simulink model "sUASTrajectoryStates"  (R2021b)
settings: Solver=VariableStepAuto  StartTime=0.0  StopTime=900  RelTol=1e-3
InitFcn:
  | FidelityStage = 2;
model workspace (MAT data in the model file):
  AirspeedVal = 58.2251893932
  LookaheadDc = 50
  LookaheadDistance = 500
  Waypoints = [-5313.43403732 -5313.49765579 -5315.24259606 -5316.98751886 -5318.73267892 -5320.47705726 -5322.22141779 -5323.96550555 -5324.69997396 -5326.29075872 -5327.88101514 -5329.47150848 ... (2598 elements, 866x3)]
  airspeedVal = 34.4977795798
  headingAngles : timeseries (value not decoded)
  lookaheadPoint : timeseries (value not decoded)
  waypointData = [-1625.03275672 -1598.86938118 -1571.45340762 -1543.27035087 -1514.50729286 -1485.12594864 -1455.09042939 -1424.58849905 -1393.84251756 -1362.78862848 -1331.63098268 -1300.4045263 ... (291 elements, 97x3)]
undefined symbols (not defined in the file): aircraftTmax, ap, DiscIntNeverNeededParam, Earth, env, initialThrottle, midFidelityUAV, sensors, trimT, uavParam, WGS84
libraries: simulink x21, mbdriLib x20, aerolibconvert2 x2, aerolibtransform2 x1, uavalgslib x1
(part 2 of 3)

== system sUASTrajectoryStates/Heading to Bank Angle ==
  TargetHeading : Inport  OutDataTypeStr=double  PortDimensions=1
  Environment : Inport  Port=2
  State : Inport  Port=3
  Bus Selector : BusSelector  OutputSignals=AirSpeed,HeadingAngle,FlightPathAngle
  Bus Selector1 : BusSelector  OutputSignals=WindNorth,WindEast,WindDown,Gravity
  HeadingControllerGain : Constant  Value=4.88135593220339  SampleTime=0.1
  Limit Bank to +- 45 deg : Saturate  UpperLimit=midFidelityUAV.maxroll/180*pi  LowerLimit=-midFidelityUAV.maxroll/180*pi
  MATLAB Function : MATLAB Function  TreatAsAtomicUnit=on
  TargetMu : Outport
  wires:
  Limit Bank to +- 45 deg/1 -> TargetMu/1  "BankAngle"
  Bus Selector1/4 -> MATLAB Function/8(Gravity)  "<Gravity>"
  Bus Selector1/3 -> MATLAB Function/7(WindDown)  "<WindDown>"
  Bus Selector1/2 -> MATLAB Function/6(WindEast)  "<WindEast>"
  Bus Selector1/1 -> MATLAB Function/5(WindNorth)  "<WindNorth>"
  TargetHeading/1 -> MATLAB Function/4(TargetHeading)
  Bus Selector/2 -> MATLAB Function/2(HeadingAngle)  "<HeadingAngle>"
  Bus Selector/1 -> MATLAB Function/1(AirSpeed)  "<AirSpeed>"
  Environment/1 -> Bus Selector1/1
  State/1 -> Bus Selector/1
  HeadingControllerGain/1 -> MATLAB Function/9(PHeadingAngle)
  Bus Selector/3 -> MATLAB Function/3(FlightPathAngle)  "<FlightPathAngle>"
  MATLAB Function/1(RollAngle) -> Limit Bank to +- 45 deg/1

== system sUASTrajectoryStates/uavEnvironment ==
  note: Gravity and Density ASSUME MKS units!
  note: Steady wind vector components (m/s).
      | (WindNorth is not from the North, as in meteorology,
      | but the component in the Northerly direction.)
  Bus Creator : BusCreator  Inputs=5
  Constant1 : Constant  Value=0
  Constant2 : Constant  Value=0
  Constant3 : Constant  Value=0
  g : Constant  Value=9.8066
  rho : Constant  Value=1.225
  SteadyEnvironment : Outport  VectorParamsAs1DForOutWhenUnconnected=off
  wires:
  Constant2/1 -> Bus Creator/2  "WindEast"
  Constant3/1 -> Bus Creator/3  "WindDown"
  Constant1/1 -> Bus Creator/1  "WindNorth"
  Bus Creator/1 -> SteadyEnvironment/1
  g/1 -> Bus Creator/4  "Gravity"
  rho/1 -> Bus Creator/5  "Density"

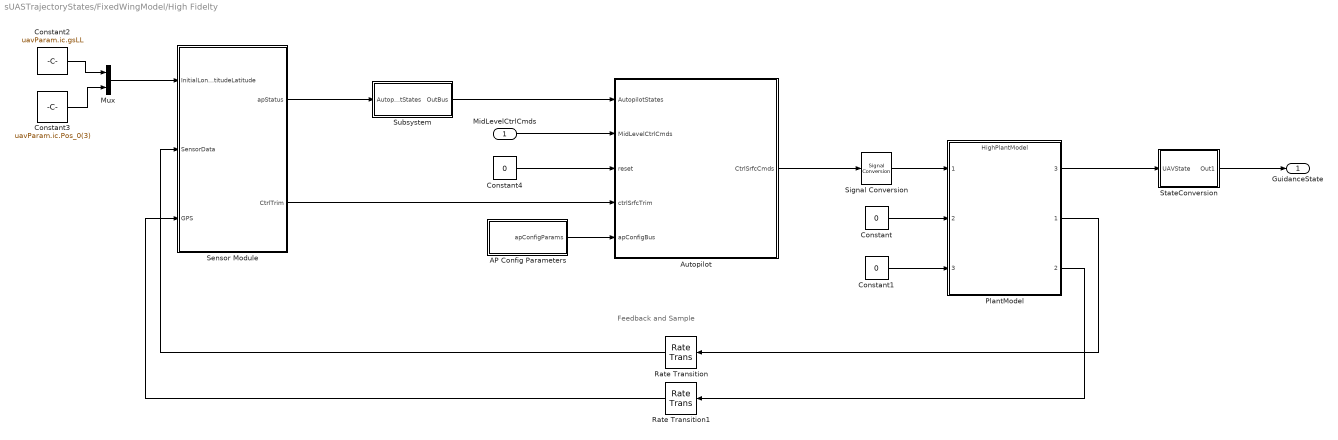
== system sUASTrajectoryStates/FixedWingModel/High Fidelty ==
  note: Feedback and Sample
  MidLevelCtrlCmds : Inport
  AP Config Parameters : Subsystem
  Autopilot : Subsystem
  Constant : Constant  Value=0
  Constant1 : Constant  Value=0
  Constant2 : Constant  Value=uavParam.ic.gsLL  OutDataTypeStr=single
  Constant3 : Constant  Value=uavParam.ic.Pos_0(3)  OutDataTypeStr=single
  Constant4 : Constant  Value=0
  Mux : Mux  Inputs=2
  PlantModel : ModelReference  ModelNameDialog=HighPlantModel.slx  SimulationMode=Normal  ModelReferenceVersion=2.0
      settings: PortSchema="{\"entries\":[{\"content\":{\"sides\":[{\"content\":{\"connectorIds\":[\"In1\",\"In2\",\"In3\"]},\"type\":\"ConnectorPlacement.EquallySpacedRectSide\",\"uuid\":\"b05064ba-762f-4c47-8c4a-e4b5b8698203\"},{\"content\":{\"connectorIds\":[\"Out3\",\"Out1\",\"Out2\"],\"side\":\"RIGHT\"},\"type\":\"ConnectorPlacement.EquallySpacedRectSide\",\"uuid\":\"4dd868b9-025c-4261-91c2-75e76041d933\"},{\"content\":{\"connectorIds\":[],\"side\":\"TOP\"},\"type\":\"ConnectorPlacement.EquallySpacedRectSide\",\"uuid\":\"bfb2a469-2e8b-4568-a482-f0d58a8ec089\"}]},\"type\":\"ConnectorPlacement.EquallySpacedConnector\",\"uuid\":\"89fe167c-302c-412e-9468-047389136680\"}],\"packageUris\":[\"http://schema.mathworks.com/mf0/Connector/R2020b\"],\"version\":\"1.0\"}"
  Rate Transition : RateTransition  OutPortSampleTime=ap.apSampleTime
  Rate Transition1 : RateTransition  OutPortSampleTime=ap.apSampleTime
      settings: AttributesFormatString=%<OutPortSampleTime>
  Sensor Module : Subsystem
  Signal Conversion : SignalConversion  ConversionOutput=Nonvirtual bus  OutDataTypeStr=Bus: ctrlCmdsBus  OverrideOpt=off
  StateConversion : Subsystem
  Subsystem : Subsystem
  GuidanceState : Outport
  wires:
  PlantModel/1 -> Rate Transition/1
  PlantModel/3 -> StateConversion/1(UAVState)
  StateConversion/1(Out1) -> GuidanceState/1
  Mux/1 -> Sensor Module/1(InitialLongtitudeLatitude)
  Constant2/1 -> Mux/1
  Constant1/1 -> PlantModel/3
  Constant/1 -> PlantModel/2
  PlantModel/2 -> Rate Transition1/1
  Constant3/1 -> Mux/2
  Rate Transition/1 -> Sensor Module/2(SensorData)
  Rate Transition1/1 -> Sensor Module/3(GPS)
  Signal Conversion/1 -> PlantModel/1
  Sensor Module/1(apStatus) -> Subsystem/1(AutopilotStates)
  Subsystem/1(OutBus) -> Autopilot/1(AutopilotStates)
  MidLevelCtrlCmds/1 -> Autopilot/2(MidLevelCtrlCmds)
  Constant4/1 -> Autopilot/3(reset)
  Sensor Module/2(CtrlTrim) -> Autopilot/4(ctrlSrfcTrim)
  AP Config Parameters/1(apConfigParams) -> Autopilot/5(apConfigBus)
  Autopilot/1(CtrlSrfcCmds) -> Signal Conversion/1

== system sUASTrajectoryStates/FixedWingModel/LowFidelity ==
  MidLevelCtrlCmds : Inport
  Bus Creator1 : BusCreator  Inputs=4  OutDataTypeStr=Bus: FixedWingEnvironmentBus  NonVirtualBus=on
  Constant : Constant  Value=0
  Constant1 : Constant  Value=0
  Constant2 : Constant  Value=0
  Constant5 : Constant  Value=env.ISA_g
  Fixed Wing UAV Guidance Model : uavalgslib/Guidance Model  ModelType=FixedWingGuidance  SpecifiedDataType=double  SimulateUsing=Code generation  InitialWorldPositionMultirotor=[0; 0; 0]  InitialWorldVelocityMultirotor=[0; 0; 0]  InitialEulerZYXMultirotor=[0; 0; 0]  InitialBodyAngularRateRPYMultirotor=[0; 0; 0]  InitialThrustMultirotor=0  InitialNorthFixedWing=0  InitialEastFixedWing=0  InitialHeightFixedWing=lowFidelityUAV.initialAltitude  InitialAirSpeedFixedWing=lowFidelityUAV.initialAirSpeed  InitialHeadingAngleFixedWing=0  InitialFlightPathAngleFixedWing=0  InitialRollAngleFixedWing=0  InitialRollAngleRateFixedWing=0  PDRollMultirotor=[3402.97,116.67]  PDPitchMultirotor=[3402.97, 116.67]  PYawRateMultirotor=1950  PThrustMultirotor=3900  MassMultirotor=0.1  PHeightFixedWing=3  PHeadingAngleFixedWing=3.9  PFlightPathAngleFixedWing=3.9  PDRollFixedWing="[5.448     4.6668]"  PAirSpeedFixedWing=7.8  FlightPathAngleLimitsFixedWing=[-pi/4, pi/4]  StateBusName='FixedWingStateBus'  ControlBusName='FixedWingControlBus'  EnvironmentBusName='FixedWingEnvironmentBus'  DataType=double
      settings: SourceProductBaseCode=UV
  GuidanceState : Outport  VectorParamsAs1DForOutWhenUnconnected=off
  wires:
  Constant5/1 -> Bus Creator1/4  "Gravity"
  Constant1/1 -> Bus Creator1/2  "WindEast"
  Bus Creator1/1 -> Fixed Wing UAV Guidance Model/2
  MidLevelCtrlCmds/1 -> Fixed Wing UAV Guidance Model/1
  Constant/1 -> Bus Creator1/1  "WindNorth"
  Fixed Wing UAV Guidance Model/1 -> GuidanceState/1
  Constant2/1 -> Bus Creator1/3  "WindDown"

== system sUASTrajectoryStates/FixedWingModel/Mid Fidelty ==
  MidLevelCtrlCmds : Inport
  Constant : Constant  Value=0
  Delay : Delay  DelayLength=1  InitialCondition=struct('Xe', [0 0 midFidelityUAV.initialAltitude], 'ias',midFidelityUAV.initialAirspeed)  SampleTime=ap.apSampleTime
  Model : ModelReference  ModelNameDialog=Outer_Loop_Autopilot.slx  SimulationMode=Normal  ModelReferenceVersion=2.10
  Rate Transition1 : RateTransition  OutPortSampleTime=0.1
  UAV Plant Dynamics : Subsystem  TreatAsAtomicUnit=on
  uavEnvironment : Subsystem  VariantControl=NoWind
  GuidanceState : Outport
  wires:
  uavEnvironment/1(SteadyEnvironment) -> UAV Plant Dynamics/2(Environment)
  Model/1 -> UAV Plant Dynamics/1(Commands)
  UAV Plant Dynamics/2(AutopilotStates) -> Rate Transition1/1
  UAV Plant Dynamics/1(uavState) -> GuidanceState/1
  Delay/1 -> Model/1
  MidLevelCtrlCmds/1 -> Model/2
  Rate Transition1/1 -> Delay/1
  Constant/1 -> Model/3

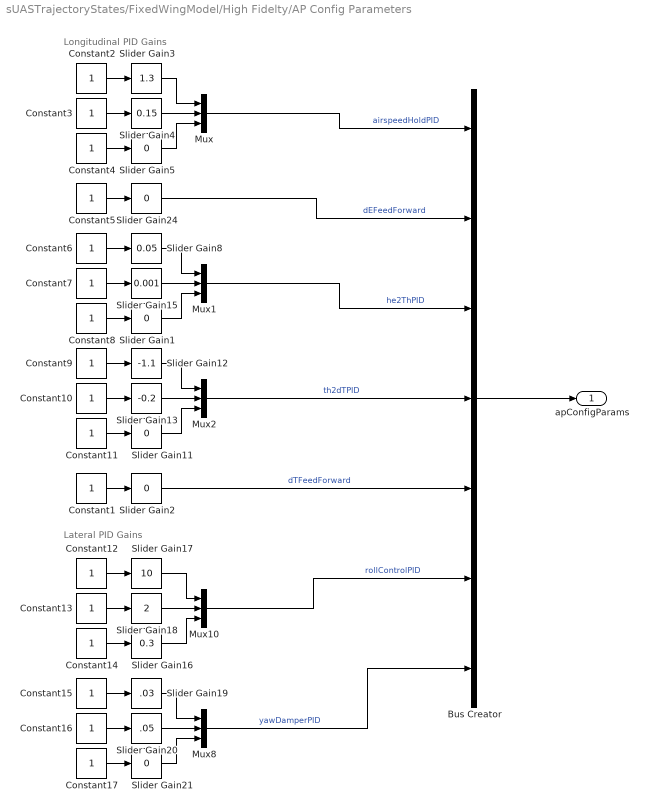
== system sUASTrajectoryStates/FixedWingModel/High Fidelty/AP Config Parameters ==
  note: Longitudinal PID Gains
  note: Lateral PID Gains
  Bus Creator : BusCreator  Inputs=7  OutDataTypeStr=Bus: apConfigParamsBus
  Constant{1..17} (17 alike) : Constant  OutDataTypeStr=single  SampleTime=ap.apSampleTime
      settings: AttributesFormatString=%<Value>
  Mux{,1..2,8,10} (5 alike) : Mux  Inputs=3
  Slider Gain1 : simulink/Math Operations/Slider Gain  gain=0  low=-20  high=20
  Slider Gain11 : simulink/Math Operations/Slider Gain  gain=0  low=-0.1  high=0
  Slider Gain12 : simulink/Math Operations/Slider Gain  gain=-1.1  low=-2  high=0.5
  Slider Gain13 : simulink/Math Operations/Slider Gain  gain=-0.2  low=-0.2  high=0
  Slider Gain15 : simulink/Math Operations/Slider Gain  gain=0.001  low=-20  high=20
  Slider Gain16 : simulink/Math Operations/Slider Gain  gain=0.3  low=-0.1  high=5
  Slider Gain17 : simulink/Math Operations/Slider Gain  gain=10  low=-0.1  high=50
  Slider Gain18 : simulink/Math Operations/Slider Gain  gain=2  low=0  high=2
  Slider Gain19 : simulink/Math Operations/Slider Gain  gain=.03  low=-20  high=20
  Slider Gain2 : simulink/Math Operations/Slider Gain  gain=0  low=-0.1  high=5
  Slider Gain20 : simulink/Math Operations/Slider Gain  gain=.05  low=-20  high=20
  Slider Gain21 : simulink/Math Operations/Slider Gain  gain=0  low=-20  high=20
  Slider Gain24 : simulink/Math Operations/Slider Gain  gain=0  low=-0.1  high=5
  Slider Gain3 : simulink/Math Operations/Slider Gain  gain=1.3  low=-0.5  high=4.5
  Slider Gain4 : simulink/Math Operations/Slider Gain  gain=0.15  low=-20  high=20
  Slider Gain5 : simulink/Math Operations/Slider Gain  gain=0  low=-20  high=20
  Slider Gain8 : simulink/Math Operations/Slider Gain  gain=0.05  low=-20  high=20
  apConfigParams : Outport  OutDataTypeStr=Bus: apConfigParamsBus  VectorParamsAs1DForOutWhenUnconnected=off
  wires:
  Mux8/1 -> Bus Creator/7  "yawDamperPID"
  Slider Gain21/1 -> Mux8/3
  Slider Gain19/1 -> Mux8/1
  Slider Gain20/1 -> Mux8/2
  Constant17/1 -> Slider Gain21/1
  Constant16/1 -> Slider Gain20/1
  Constant15/1 -> Slider Gain19/1
  Mux10/1 -> Bus Creator/6  "rollControlPID"
  Slider Gain16/1 -> Mux10/3
  Slider Gain17/1 -> Mux10/1
  Slider Gain18/1 -> Mux10/2
  Constant14/1 -> Slider Gain16/1
  Constant13/1 -> Slider Gain18/1
  Constant12/1 -> Slider Gain17/1
  Constant1/1 -> Slider Gain2/1
  Slider Gain1/1 -> Mux1/3
  Slider Gain15/1 -> Mux1/2
  Mux2/1 -> Bus Creator/4  "th2dTPID"
  Slider Gain11/1 -> Mux2/3
  Slider Gain12/1 -> Mux2/1
  Slider Gain13/1 -> Mux2/2
  Constant11/1 -> Slider Gain11/1
  Constant10/1 -> Slider Gain13/1
  Constant9/1 -> Slider Gain12/1
  Mux1/1 -> Bus Creator/3  "he2ThPID"
  Slider Gain8/1 -> Mux1/1
  Constant8/1 -> Slider Gain1/1
  Constant7/1 -> Slider Gain15/1
  Constant6/1 -> Slider Gain8/1
  Slider Gain24/1 -> Bus Creator/2  "dEFeedForward"
  Constant5/1 -> Slider Gain24/1
  Mux/1 -> Bus Creator/1  "airspeedHoldPID"
  Slider Gain5/1 -> Mux/3
  Slider Gain3/1 -> Mux/1
  Slider Gain4/1 -> Mux/2
  Constant4/1 -> Slider Gain5/1
  Constant3/1 -> Slider Gain4/1
  Constant2/1 -> Slider Gain3/1
  Bus Creator/1 -> apConfigParams/1
  Slider Gain2/1 -> Bus Creator/5  "dTFeedForward"

== system sUASTrajectoryStates/FixedWingModel/High Fidelty/Autopilot ==
  note: Signal Routing
  AutopilotStates : Inport
  MidLevelCtrlCmds : Inport  Port=2
  reset : Inport  Port=3
  ctrlSrfcTrim : Inport  Port=4
  apConfigBus : Inport  Port=5
  Inner Loop Autopilot : Subsystem
  Outer Loop Autopilot : ModelReference  ModelNameDialog=Outer_Loop_Autopilot.slx  SimulationMode=Normal  ModelReferenceVersion=2.6
      settings: PortSchema="{\"entries\":[{\"content\":{\"sides\":[{\"content\":{\"connectorIds\":[\"In2\",\"In1\",\"In3\"]},\"type\":\"ConnectorPlacement.EquallySpacedRectSide\",\"uuid\":\"ffbe0e68-5eaf-4f2c-bade-2815524b0984\"},{\"content\":{\"connectorIds\":[\"Out1\"],\"side\":\"RIGHT\"},\"type\":\"ConnectorPlacement.EquallySpacedRectSide\",\"uuid\":\"57fe3717-6620-4a33-be9b-5bc5f2cad269\"},{\"content\":{\"connectorIds\":[],\"side\":\"TOP\"},\"type\":\"ConnectorPlacement.EquallySpacedRectSide\",\"uuid\":\"35a1b882-87be-41ec-998f-2c84a3803ec5\"}]},\"type\":\"ConnectorPlacement.EquallySpacedConnector\",\"uuid\":\"d728f9c7-d9da-4786-9d89-76839d7f2fee\"}],\"packageUris\":[\"http://schema.mathworks.com/mf0/Connector/R2020b\"],\"version\":\"1.0\"}"
  CtrlSrfcCmds : Outport
  wires:
  Inner Loop Autopilot/1(CtrlSrfcCmds) -> CtrlSrfcCmds/1
  [AutopilotStates] -> Outer Loop Autopilot/1
  MidLevelCtrlCmds/1 -> Outer Loop Autopilot/2
  apConfigBus/1 -> Inner Loop Autopilot/5(apConfigBus)
  Outer Loop Autopilot/1 -> Inner Loop Autopilot/1(LowLevelCtrlCmds)
  ctrlSrfcTrim/1 -> Inner Loop Autopilot/4(ctrlSrfcTrim)
  AutopilotStates/1 -> [AutopilotStates]
  reset/1 -> [reset]
  [AutopilotStates] -> Inner Loop Autopilot/2(AutopilotStates)
  [reset] -> Inner Loop Autopilot/3(reset)
  [reset] -> Outer Loop Autopilot/3

== system sUASTrajectoryStates/FixedWingModel/High Fidelty/Sensor Module ==
  InitialLongtitudeLatitude : Inport
  SensorData : Inport  Port=2
  GPS : Inport  Port=3
  Position Filter : Subsystem  TreatAsAtomicUnit=on
  SensorConditioning : Subsystem  TreatAsAtomicUnit=on
  apStatusCreation : Subsystem
  apStatus : Outport  VectorParamsAs1DForOutWhenUnconnected=off
  CtrlTrim : Outport  Port=2  VectorParamsAs1DForOutWhenUnconnected=off
  wires:
  InitialLongtitudeLatitude/1 -> Position Filter/3(InitialLongtitudeLatitude)
  SensorConditioning/1(FilteredSensorData) -> apStatusCreation/3(FilteredSensorData), Position Filter/1(FilteredSensorData)
  SensorConditioning/2(CtrlSurfaces) -> CtrlTrim/1
  GPS/1 -> apStatusCreation/2(GPSData), Position Filter/2(GPSData)
  SensorData/1 -> SensorConditioning/1(RawSensorData)
  apStatusCreation/1(apStatus) -> apStatus/1
  Position Filter/1(PosVel_hat) -> apStatusCreation/1(PosVel_hat)

== system sUASTrajectoryStates/FixedWingModel/High Fidelty/StateConversion ==
  UAVState : Inport
  Bus Creator : BusCreator  Inputs=8  OutDataTypeStr=Bus: FixedWingStateBus  NonVirtualBus=on
  Bus Selector : BusSelector  OutputSignals=X_e,airspeed,V_e,Euler,pqr
  Demux : Demux  Outputs=3
  Gain : Gain  Gain=-1
  Gain1 : Gain
  Selector : Selector  InputPortWidth=3  IndexOptions=Index vector (dialog)  Indices=[1]  OutputSizes=1
  Selector1 : Selector  InputPortWidth=3  IndexOptions=Index vector (dialog)  Indices=[1]  OutputSizes=1
  Subsystem : Subsystem
  Out1 : Outport  VectorParamsAs1DForOutWhenUnconnected=off
  wires:
  Bus Creator/1 -> Out1/1
  Gain1/1 -> Bus Creator/4  "AirSpeed"
  Subsystem/2(FlightPath) -> Bus Creator/6  "FlightPathAngle"
  Bus Selector/2 -> Gain1/1  "<airspeed>"
  Selector/1 -> Bus Creator/7  "RollAngle"
  Bus Selector/4 -> Selector/1  "<Euler>"
  Bus Selector/1 -> Demux/1  "<X_e>"
  Bus Selector/3 -> Subsystem/1(Ve)  "<V_e>"
  Demux/2 -> Bus Creator/2  "East"
  Bus Selector/5 -> Selector1/1  "<pqr>"
  Subsystem/1(Heading) -> Bus Creator/5  "HeadingAngle"
  Demux/1 -> Bus Creator/1  "North"
  Demux/3 -> Gain/1
  Selector1/1 -> Bus Creator/8  "RollAngleRate"
  Gain/1 -> Bus Creator/3  "Height"
  UAVState/1 -> Bus Selector/1

== system sUASTrajectoryStates/FixedWingModel/High Fidelty/Subsystem ==
  In Bus Element : Inport  PortName=AutopilotStates  Element=Ab
  In Bus Element2 : Inport  PortName=AutopilotStates  Element=Euler
  In Bus Element5 : Inport  PortName=AutopilotStates  Element=Xe
  In Bus Element4 : Inport  PortName=AutopilotStates  Element=ias
  Data Type Conversion{,2..3,5} (4 alike) : DataTypeConversion  OutDataTypeStr=double
  Out Bus Element : Outport  PortName=OutBus  Element=Ab
  Out Bus Element2 : Outport  PortName=OutBus  Element=Euler
  Out Bus Element4 : Outport  PortName=OutBus  Element=Xe
  Out Bus Element7 : Outport  PortName=OutBus  Element=ias
  wires:
  In Bus Element4/1 -> Data Type Conversion3/1  "ias"
  In Bus Element5/1 -> Data Type Conversion5/1  "Xe"
  In Bus Element2/1 -> Data Type Conversion2/1  "Euler"
  In Bus Element/1 -> Data Type Conversion/1  "Ab"
  Data Type Conversion/1 -> Out Bus Element/1
  Data Type Conversion2/1 -> Out Bus Element2/1
  Data Type Conversion3/1 -> Out Bus Element7/1
  Data Type Conversion5/1 -> Out Bus Element4/1

== system sUASTrajectoryStates/FixedWingModel/Mid Fidelty/UAV Plant Dynamics ==
  Commands : Inport
  Environment : Inport  Port=2
  Vehicle Dynamics : Subsystem
  asbState to uavState : Subsystem
  uavState : Outport
  AutopilotStates : Outport  Port=2
  wires:
  Vehicle Dynamics/1(AutopilotState) -> asbState to uavState/1(asbState), AutopilotStates/1
  asbState to uavState/1(uavState) -> uavState/1
  Commands/1 -> Vehicle Dynamics/1(Commands)
  Environment/1 -> Vehicle Dynamics/2(Environment)

== system sUASTrajectoryStates/FixedWingModel/Mid Fidelty/uavEnvironment ==
  note: Gravity and Density ASSUME MKS units!
  note: Steady wind vector components (m/s).
      | (WindNorth is not from the North, as in meteorology,
      | but the component in the Northerly direction.)
  Bus Creator : BusCreator  Inputs=5
  Constant1 : Constant  Value=0
  Constant2 : Constant  Value=0
  Constant3 : Constant  Value=0
  g : Constant  Value=9.8066
  rho : Constant  Value=1.225
  SteadyEnvironment : Outport  VectorParamsAs1DForOutWhenUnconnected=off
  wires:
  Constant2/1 -> Bus Creator/2  "WindEast"
  Constant3/1 -> Bus Creator/3  "WindDown"
  Constant1/1 -> Bus Creator/1  "WindNorth"
  Bus Creator/1 -> SteadyEnvironment/1
  g/1 -> Bus Creator/4  "Gravity"
  rho/1 -> Bus Creator/5  "Density"

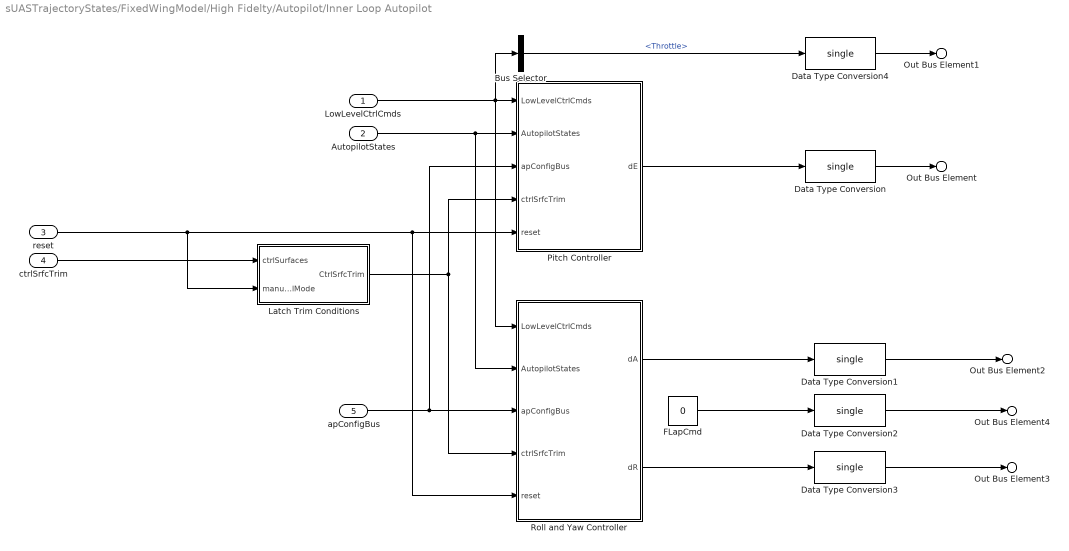
== system sUASTrajectoryStates/FixedWingModel/High Fidelty/Autopilot/Inner Loop Autopilot ==
  LowLevelCtrlCmds : Inport
  AutopilotStates : Inport  Port=2
  reset : Inport  Port=3
  ctrlSrfcTrim : Inport  Port=4
  apConfigBus : Inport  Port=5
  Bus Selector : BusSelector  OutputSignals=Throttle
  Data Type Conversion{,1..4} (5 alike) : DataTypeConversion  OutDataTypeStr=single
  FLapCmd : Constant  Value=0  OutDataTypeStr=single  SampleTime=ap.apSampleTime
      settings: AttributesFormatString=%<Value>
  Latch Trim Conditions : Subsystem
  Pitch Controller : Subsystem  VariantControl=AltCont==0
  Roll and Yaw Controller : Subsystem  TreatAsAtomicUnit=on
  Out Bus Element : Outport  PortName=CtrlSrfcCmds  Element=elevatorCmd
  Out Bus Element1 : Outport  PortName=CtrlSrfcCmds  Element=throttleCmd
  Out Bus Element2 : Outport  PortName=CtrlSrfcCmds  Element=aileronCmd
  Out Bus Element3 : Outport  PortName=CtrlSrfcCmds  Element=rudderCmd
  Out Bus Element4 : Outport  PortName=CtrlSrfcCmds  Element=flapCmd
  wires:
  Pitch Controller/1(dE) -> Data Type Conversion/1
  LowLevelCtrlCmds/1 -> Bus Selector/1, Roll and Yaw Controller/1(LowLevelCtrlCmds), Pitch Controller/1(LowLevelCtrlCmds)
  AutopilotStates/1 -> Roll and Yaw Controller/2(AutopilotStates), Pitch Controller/2(AutopilotStates)
  Latch Trim Conditions/1(CtrlSrfcTrim) -> Roll and Yaw Controller/4(ctrlSrfcTrim), Pitch Controller/4(ctrlSrfcTrim)
  Roll and Yaw Controller/1(dA) -> Data Type Conversion1/1
  Roll and Yaw Controller/2(dR) -> Data Type Conversion3/1
  apConfigBus/1 -> Pitch Controller/3(apConfigBus), Roll and Yaw Controller/3(apConfigBus)
  Bus Selector/1 -> Data Type Conversion4/1  "<Throttle>"
  ctrlSrfcTrim/1 -> Latch Trim Conditions/1(ctrlSurfaces)
  reset/1 -> Latch Trim Conditions/2(manualMode), Roll and Yaw Controller/5(reset), Pitch Controller/5(reset)
  Data Type Conversion/1 -> Out Bus Element/1
  Data Type Conversion1/1 -> Out Bus Element2/1
  FLapCmd/1 -> Data Type Conversion2/1
  Data Type Conversion2/1 -> Out Bus Element4/1
  Data Type Conversion3/1 -> Out Bus Element3/1
  Data Type Conversion4/1 -> Out Bus Element1/1

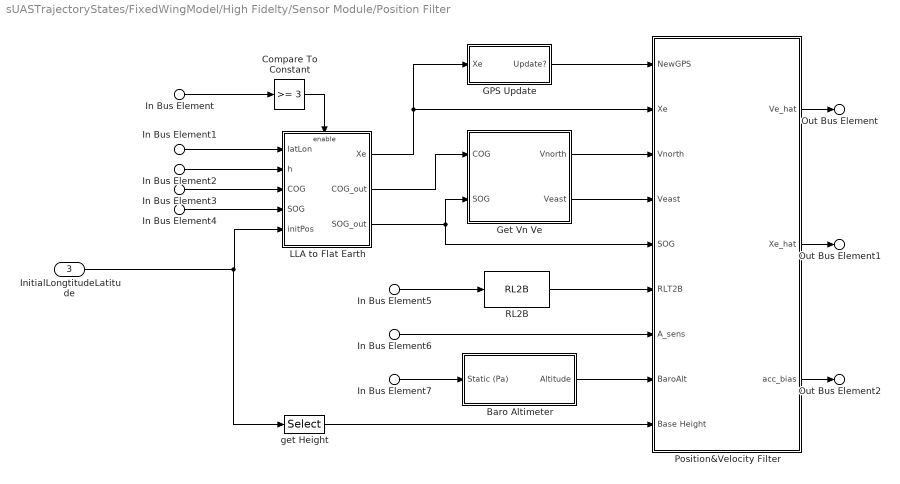
== system sUASTrajectoryStates/FixedWingModel/High Fidelty/Sensor Module/Position Filter ==
  In Bus Element5 : Inport  PortName=FilteredSensorData  Element=Euler
  In Bus Element6 : Inport  PortName=FilteredSensorData  Element=Ab
  In Bus Element7 : Inport  PortName=FilteredSensorData  Element=baro
  In Bus Element : Inport  Port=2  PortName=GPSData  Element=gps_fix
  In Bus Element1 : Inport  Port=2  PortName=GPSData  Element=gps_latLon
  In Bus Element2 : Inport  Port=2  PortName=GPSData  Element=gps_h
  In Bus Element3 : Inport  Port=2  PortName=GPSData  Element=gps_cog
  In Bus Element4 : Inport  Port=2  PortName=GPSData  Element=gps_sog
  InitialLongtitudeLatitude : Inport  Port=3
  Baro Altimeter : Subsystem
  Compare To Constant : simulink/Logic and Bit Operations/Compare To Constant  relop=>=  const=3  OutDataTypeStr=boolean
  GPS Update : Subsystem  mask{T=ap.apSampleTime}
      mask prompts: T "Sample Time"
  Get Vn Ve : Subsystem
  LLA to Flat Earth : Subsystem
  Position&Velocity Filter : Subsystem
  RL2B : mbdriLib/Coordinates/RL2B  SystemSampleTime=-1  VariantActivationTime=update diagram  Latency=0  AutoFrameSizeCalculation=off
  get Height : Selector  InputPortWidth=3  IndexOptions=Index vector (dialog)  Indices=[3]  OutputSizes=1
  Out Bus Element : Outport  VectorParamsAs1DForOutWhenUnconnected=off  PortName=PosVel_hat  Element=Ve_hat
  Out Bus Element1 : Outport  VectorParamsAs1DForOutWhenUnconnected=off  PortName=PosVel_hat  Element=Xe_hat
  Out Bus Element2 : Outport  VectorParamsAs1DForOutWhenUnconnected=off  PortName=PosVel_hat  Element=Ab_bias_hat
  wires:
  LLA to Flat Earth/1(Xe) -> Position&Velocity Filter/2(Xe), GPS Update/1(Xe)
  get Height/1 -> Position&Velocity Filter/9(Base Height)
  In Bus Element6/1 -> Position&Velocity Filter/7(A_sens)
  RL2B/1 -> Position&Velocity Filter/6(RLT2B)
  In Bus Element5/1 -> RL2B/1
  In Bus Element7/1 -> Baro Altimeter/1(Static (Pa))
  Baro Altimeter/1(Altitude) -> Position&Velocity Filter/8(BaroAlt)
  Get Vn Ve/2(Veast) -> Position&Velocity Filter/4(Veast)
  Get Vn Ve/1(Vnorth) -> Position&Velocity Filter/3(Vnorth)
  GPS Update/1(Update?) -> Position&Velocity Filter/1(NewGPS)
  InitialLongtitudeLatitude/1 -> LLA to Flat Earth/5(initPos), get Height/1
  In Bus Element4/1 -> LLA to Flat Earth/4(SOG)
  In Bus Element3/1 -> LLA to Flat Earth/3(COG)
  In Bus Element2/1 -> LLA to Flat Earth/2(h)
  In Bus Element1/1 -> LLA to Flat Earth/1(latLon)
  Compare To Constant/1 -> LLA to Flat Earth/Enable
  In Bus Element/1 -> Compare To Constant/1
  Position&Velocity Filter/2(Xe_hat) -> Out Bus Element1/1
  Position&Velocity Filter/1(Ve_hat) -> Out Bus Element/1
  Position&Velocity Filter/3(acc_bias) -> Out Bus Element2/1
  LLA to Flat Earth/2(COG_out) -> Get Vn Ve/1(COG)
  LLA to Flat Earth/3(SOG_out) -> Get Vn Ve/2(SOG), Position&Velocity Filter/5(SOG)

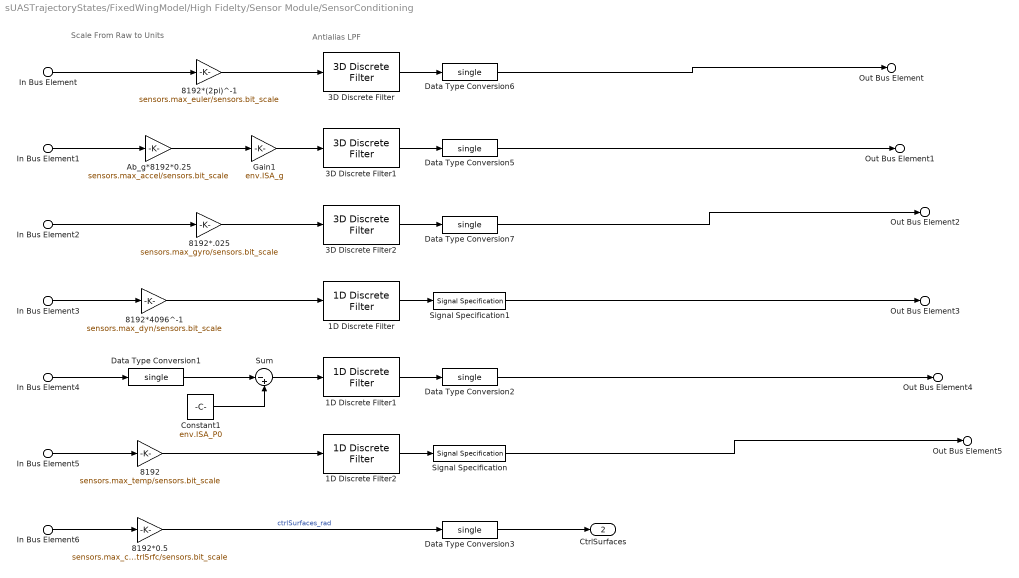
== system sUASTrajectoryStates/FixedWingModel/High Fidelty/Sensor Module/SensorConditioning ==
  note: Antialias LPF
  note: Scale From Raw to Units
  In Bus Element : Inport  PortName=RawSensorData  Element=Euler_raw
  In Bus Element1 : Inport  PortName=RawSensorData  Element=Ab_raw
  In Bus Element2 : Inport  PortName=RawSensorData  Element=G_raw
  In Bus Element3 : Inport  PortName=RawSensorData  Element=q_raw
  In Bus Element4 : Inport  PortName=RawSensorData  Element=static_raw
  In Bus Element5 : Inport  PortName=RawSensorData  Element=T_raw
  In Bus Element6 : Inport  PortName=RawSensorData  Element=ctrlSurface_PWM
  1D Discrete Filter : mbdriLib/Filtering/1D Discrete Filter  bw=sensors.antialiasBW  TSample=ap.apSampleTime
      settings: AttributesFormatString=Fc = 40
  1D Discrete Filter1 : mbdriLib/Filtering/1D Discrete Filter  bw=sensors.antialiasBW  TSample=ap.apSampleTime
      settings: AttributesFormatString=Fc = 40
  1D Discrete Filter2 : mbdriLib/Filtering/1D Discrete Filter  bw=sensors.antialiasBW  TSample=ap.apSampleTime
      settings: AttributesFormatString=Fc = 40
  3D Discrete Filter : mbdriLib/Filtering/3D Discrete Filter  bw=sensors.antialiasBW  TSample=ap.apSampleTime
      settings: AttributesFormatString=Fc = 40
  3D Discrete Filter1 : mbdriLib/Filtering/3D Discrete Filter  bw=sensors.antialiasBW  TSample=ap.apSampleTime
      settings: AttributesFormatString=Fc = 40
  3D Discrete Filter2 : mbdriLib/Filtering/3D Discrete Filter  bw=sensors.antialiasBW  TSample=ap.apSampleTime
      settings: AttributesFormatString=Fc = 40
  8192 : Gain  Description=8192/1  Gain=sensors.max_temp/sensors.bit_scale  OutDataTypeStr=single
      settings: AttributesFormatString=%<Gain>
  8192*(2pi)^-1 : Gain  Gain=sensors.max_euler/sensors.bit_scale  OutDataTypeStr=single
      settings: AttributesFormatString=%<Gain>
  8192*.025 : Gain  Gain=sensors.max_gyro/sensors.bit_scale  OutDataTypeStr=single
      settings: AttributesFormatString=%<Gain>
  8192*0.5 : Gain  Gain=sensors.max_ctrlSrfc/sensors.bit_scale  OutDataTypeStr=single
      settings: AttributesFormatString=%<Gain>
  8192*4096^-1 : Gain  Gain=sensors.max_dyn/sensors.bit_scale  OutDataTypeStr=single
      settings: AttributesFormatString=%<Gain>
  Ab_g*8192*0.25 : Gain  Gain=sensors.max_accel/sensors.bit_scale  OutDataTypeStr=single
      settings: AttributesFormatString=%<Gain>
  Constant1 : Constant  Value=env.ISA_P0
      settings: AttributesFormatString=%<Value>
  Data Type Conversion{1..3,5..7} (6 alike) : DataTypeConversion  OutDataTypeStr=single
  Gain1 : Gain  Gain=env.ISA_g  OutDataTypeStr=single
      settings: AttributesFormatString=%<Gain>
  Signal Specification : SignalSpecification  OutDataTypeStr=single  Unit=K
  Signal Specification1 : SignalSpecification  OutDataTypeStr=single  Unit=Pa
  Sum : Sum  Inputs=|-+
  Out Bus Element : Outport  VectorParamsAs1DForOutWhenUnconnected=off  PortName=FilteredSensorData  Element=Euler
  Out Bus Element1 : Outport  VectorParamsAs1DForOutWhenUnconnected=off  PortName=FilteredSensorData  Element=Ab
  Out Bus Element2 : Outport  VectorParamsAs1DForOutWhenUnconnected=off  PortName=FilteredSensorData  Element=G
  Out Bus Element3 : Outport  VectorParamsAs1DForOutWhenUnconnected=off  PortName=FilteredSensorData  Element=q
  Out Bus Element4 : Outport  VectorParamsAs1DForOutWhenUnconnected=off  PortName=FilteredSensorData  Element=baro
  Out Bus Element5 : Outport  VectorParamsAs1DForOutWhenUnconnected=off  PortName=FilteredSensorData  Element=T
  CtrlSurfaces : Outport  Port=2  VectorParamsAs1DForOutWhenUnconnected=off
  wires:
  8192*0.5/1 -> Data Type Conversion3/1  "ctrlSurfaces_rad"
  In Bus Element6/1 -> 8192*0.5/1
  Data Type Conversion3/1 -> CtrlSurfaces/1
  1D Discrete Filter2/1 -> Signal Specification/1
  Data Type Conversion2/1 -> Out Bus Element4/1
  1D Discrete Filter1/1 -> Data Type Conversion2/1
  1D Discrete Filter/1 -> Signal Specification1/1
  3D Discrete Filter2/1 -> Data Type Conversion7/1
  3D Discrete Filter1/1 -> Data Type Conversion5/1
  3D Discrete Filter/1 -> Data Type Conversion6/1
  Data Type Conversion1/1 -> Sum/1
  Gain1/1 -> 3D Discrete Filter1/1
  In Bus Element1/1 -> Ab_g*8192*0.25/1
  Data Type Conversion6/1 -> Out Bus Element/1
  Data Type Conversion5/1 -> Out Bus Element1/1
  Data Type Conversion7/1 -> Out Bus Element2/1
  Signal Specification1/1 -> Out Bus Element3/1
  Sum/1 -> 1D Discrete Filter1/1
  Signal Specification/1 -> Out Bus Element5/1
  Constant1/1 -> Sum/2
  8192/1 -> 1D Discrete Filter2/1
  8192*4096^-1/1 -> 1D Discrete Filter/1
  In Bus Element5/1 -> 8192/1
  In Bus Element4/1 -> Data Type Conversion1/1
  In Bus Element3/1 -> 8192*4096^-1/1
  In Bus Element2/1 -> 8192*.025/1
  8192*.025/1 -> 3D Discrete Filter2/1
  8192*(2pi)^-1/1 -> 3D Discrete Filter/1
  Ab_g*8192*0.25/1 -> Gain1/1
  In Bus Element/1 -> 8192*(2pi)^-1/1

== system sUASTrajectoryStates/FixedWingModel/High Fidelty/Sensor Module/apStatusCreation ==
  In Bus Element7 : Inport  PortName=PosVel_hat  Element=Xe_hat
  In Bus Element8 : Inport  PortName=PosVel_hat  Element=Ve_hat
  In Bus Element10 : Inport  Port=2  PortName=GPSData
  In Bus Element9 : Inport  Port=2  PortName=GPSData  Element=gps_h
  In Bus Element : Inport  Port=3  PortName=FilteredSensorData  Element=Ab
  In Bus Element1 : Inport  Port=3  PortName=FilteredSensorData  Element=G
  In Bus Element2 : Inport  Port=3  PortName=FilteredSensorData  Element=Euler
  In Bus Element3 : Inport  Port=3  PortName=FilteredSensorData  Element=baro
  In Bus Element4 : Inport  Port=3  PortName=FilteredSensorData  Element=q
  Air Density from Height : mbdriLib/Air Utilities/Air Density from Height  SystemSampleTime=-1  VariantActivationTime=update diagram  Latency=0  AutoFrameSizeCalculation=off
  Bus Creator1 : BusCreator  Inputs=8  OutDataTypeStr=Bus: apStatusBus  NonVirtualBus=on
  Compute Airspeed : mbdriLib/Air Utilities/Compute Airspeed  SystemSampleTime=-1  VariantActivationTime=update diagram  Latency=0  AutoFrameSizeCalculation=off
  apStatus : Outport  VectorParamsAs1DForOutWhenUnconnected=off
  wires:
  In Bus Element1/1 -> Bus Creator1/2  "G"
  In Bus Element/1 -> Bus Creator1/1  "Ab"
  In Bus Element10/1 -> Bus Creator1/8  "GPS"
  In Bus Element2/1 -> Bus Creator1/3  "Euler"
  Compute Airspeed/1 -> Bus Creator1/4  "ias"
  Air Density from Height/1 -> Compute Airspeed/2
  In Bus Element8/1 -> Bus Creator1/7  "Ve"
  Bus Creator1/1 -> apStatus/1
  In Bus Element4/1 -> Compute Airspeed/1
  In Bus Element3/1 -> Bus Creator1/5  "baro"
  In Bus Element7/1 -> Bus Creator1/6  "Xe"
  In Bus Element9/1 -> Air Density from Height/1

== system sUASTrajectoryStates/FixedWingModel/High Fidelty/StateConversion/Subsystem ==
  Ve : Inport
  Add : Sum
  Atan : Trigonometry  Operator=atan2
  Atan1 : Trigonometry  Operator=atan2
  Demux : Demux  Outputs=2
  Selector : Selector  InputPortWidth=3  IndexOptions=Index vector (dialog)  Indices=[2 1]  OutputSizes=1
  Selector1 : Selector  InputPortWidth=3  IndexOptions=Index vector (dialog)  Indices=[3]  OutputSizes=1
  Sqrt : Sqrt  SaturateOnIntegerOverflow=on
  Square : Math  Operator=square  SignedPower=on  SaturateOnIntegerOverflow=on
  Square1 : Math  Operator=square  SignedPower=on  SaturateOnIntegerOverflow=on
  Heading : Outport  VectorParamsAs1DForOutWhenUnconnected=off
  FlightPath : Outport  Port=2  VectorParamsAs1DForOutWhenUnconnected=off
  wires:
  Demux/1 -> Square/1, Atan/1
  Demux/2 -> Square1/1, Atan/2
  Selector/1 -> Demux/1
  Ve/1 -> Selector1/1, Selector/1
  Atan/1 -> Heading/1
  Atan1/1 -> FlightPath/1
  Selector1/1 -> Atan1/1
  Add/1 -> Sqrt/1
  Sqrt/1 -> Atan1/2
  Square/1 -> Add/1
  Square1/1 -> Add/2

== system sUASTrajectoryStates/FixedWingModel/Mid Fidelty/UAV Plant Dynamics/Vehicle Dynamics ==
  Commands : Inport
  Environment : Inport  Port=2
  AutopilotStates : Subsystem
  Calculate Forces : Subsystem
  Feedback : Subsystem
  Fixed-Wing UAV Point Mass : UAVPointMass  east=midFidelityUAV.initialEast  north=midFidelityUAV.initialNorth  altitude=midFidelityUAV.initialAltitude  airspeed=midFidelityUAV.initialAirspeed  gamma=midFidelityUAV.initialFlightPathAngle  chi=midFidelityUAV.initialHeadingAngle  mass=midFidelityUAV.aircraftM
  AutopilotState : Outport
  wires:
  Calculate Forces/5(gamma_a) -> Fixed-Wing UAV Point Mass/5
  Commands/1 -> Calculate Forces/2(Cmds)
  Calculate Forces/1(Lift) -> Fixed-Wing UAV Point Mass/1
  Feedback/1(Feedback) -> Calculate Forces/1(Feedback)
  AutopilotStates/1(AutopilotStates) -> Feedback/1(AutopilotStates), AutopilotState/1
  Fixed-Wing UAV Point Mass/1 -> AutopilotStates/1(V)
  Fixed-Wing UAV Point Mass/2 -> AutopilotStates/2(G)
  Fixed-Wing UAV Point Mass/3 -> AutopilotStates/3(Va)
  Fixed-Wing UAV Point Mass/4 -> AutopilotStates/4(Ve)
  Fixed-Wing UAV Point Mass/5 -> AutopilotStates/5(XNED)
  Fixed-Wing UAV Point Mass/6 -> AutopilotStates/6(gam_a)
  Fixed-Wing UAV Point Mass/7 -> AutopilotStates/7(gam)
  Fixed-Wing UAV Point Mass/8 -> AutopilotStates/8(chi_a)
  Environment/1 -> Calculate Forces/3(Environment)
  Calculate Forces/2(Drag) -> Fixed-Wing UAV Point Mass/2
  Calculate Forces/3(Weight1) -> Fixed-Wing UAV Point Mass/3
  Calculate Forces/4(Thrust1) -> Fixed-Wing UAV Point Mass/4
  Calculate Forces/6(mu) -> Fixed-Wing UAV Point Mass/6, AutopilotStates/10(mu)
  Calculate Forces/8(WindVector) -> Fixed-Wing UAV Point Mass/8
  Calculate Forces/7(alpha) -> Fixed-Wing UAV Point Mass/7
  Fixed-Wing UAV Point Mass/9 -> AutopilotStates/9(chi)

== system sUASTrajectoryStates/FixedWingModel/Mid Fidelty/UAV Plant Dynamics/asbState to uavState ==
  note: Convert from the ASB State to the UAV Robotics State.
  asbState : Inport
  Bus Creator : BusCreator  Inputs=8
  Bus Selector : BusSelector  OutputSignals=Xe,Va,chi,gamma,mu
  Rename chi : Subsystem
  Rename gamma : Subsystem
  Rename mu : Subsystem
  Roll rate Do not use : Constant  Value=0  SampleTime=0.1
  Select East : Selector  InputPortWidth=3  IndexOptions=Index vector (dialog)  Indices=[2]  OutputSizes=1
  Select Height : Selector  InputPortWidth=3  IndexOptions=Index vector (dialog)  Indices=[3]  OutputSizes=1
  Select North : Selector  InputPortWidth=3  IndexOptions=Index vector (dialog)  Indices=[1]  OutputSizes=1
  Vector Length : Subsystem
  uavState : Outport
  wires:
  Bus Selector/3 -> Rename chi/1(In1)  "<chi>"
  Bus Selector/4 -> Rename gamma/1(In1)  "<gamma>"
  Bus Selector/5 -> Rename mu/1(In1)  "<mu>"
  asbState/1 -> Bus Selector/1
  Bus Creator/1 -> uavState/1
  Bus Selector/1 -> Select Height/1, Select East/1, Select North/1  "<Xe>"
  Select East/1 -> Bus Creator/2  "East"
  Select North/1 -> Bus Creator/1  "North"
  Select Height/1 -> Bus Creator/3  "Height"
  Bus Selector/2 -> Vector Length/1(3DVector)  "<Va>"
  Vector Length/1(norm) -> Bus Creator/4  "AirSpeed"
  Rename gamma/1(Out1) -> Bus Creator/6  "FlightPathAngle"
  Rename chi/1(Out1) -> Bus Creator/5  "HeadingAngle"
  Rename mu/1(Out1) -> Bus Creator/7  "RollAngle"
  Roll rate Do not use/1 -> Bus Creator/8  "RollAngleRate"

== system sUASTrajectoryStates/FixedWingModel/High Fidelty/Autopilot/Inner Loop Autopilot/Latch Trim Conditions ==
  ctrlSurfaces : Inport
  manualMode : Inport  Port=2
  Compare To Constant : simulink/Logic and Bit Operations/Compare To Constant  relop===  const=1  OutDataTypeStr=boolean
  Latch Control Surfaces Trim from any mode : Subsystem  TreatAsAtomicUnit=on
  CtrlSrfcTrim : Outport  VectorParamsAs1DForOutWhenUnconnected=off
  wires:
  manualMode/1 -> Compare To Constant/1
  Latch Control Surfaces Trim from any mode/1(Trim) -> CtrlSrfcTrim/1
  Compare To Constant/1 -> Latch Control Surfaces Trim from any mode/Trigger
  ctrlSurfaces/1 -> Latch Control Surfaces Trim from any mode/1(ctrlSurfaces)

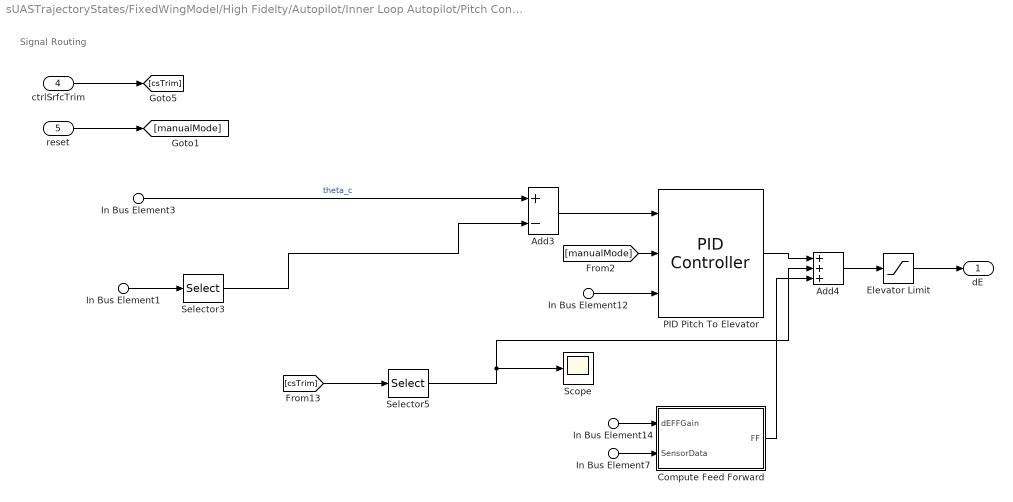
== system sUASTrajectoryStates/FixedWingModel/High Fidelty/Autopilot/Inner Loop Autopilot/Pitch Controller ==
  note: Signal Routing
  In Bus Element3 : Inport  PortName=LowLevelCtrlCmds  Element=Pitch
  In Bus Element7 : Inport  Port=2  PortName=AutopilotStates
  In Bus Element1 : Inport  Port=2  PortName=AutopilotStates  Element=Euler
  In Bus Element12 : Inport  Port=3  PortName=apConfigBus  Element=th2dTPID
  In Bus Element14 : Inport  Port=3  PortName=apConfigBus  Element=dTFeedForward
  ctrlSrfcTrim : Inport  Port=4
  reset : Inport  Port=5
  Add3 : Sum  Inputs=+-  OutDataTypeStr=single
  Add4 : Sum  Inputs=3  OutDataTypeStr=single
  Compute Feed Forward : Subsystem
  Elevator Limit : Saturate  UpperLimit=ap.control.deLimit  LowerLimit=-ap.control.deLimit
      settings: AttributesFormatString="[%<LowerLimit>  %<UpperLimit>]"
  PID Pitch To Elevator : mbdriLib/Control/PID Controller  Tsample=ap.apSampleTime  Ndelay=ap.control.derivativesConstant  upperSaturationLimit=ap.control.deLimit  lowerSaturationLimit=-ap.control.deLimit
  Scope : Scope
  Selector3 : Selector  InputPortWidth=3  IndexOptions=Index vector (dialog)  Indices=[2]  OutputSizes=1
  Selector5 : Selector  InputPortWidth=5  IndexOptions=Index vector (dialog)  Indices=[5]  OutputSizes=1
  dE : Outport  VectorParamsAs1DForOutWhenUnconnected=off
  wires:
  In Bus Element3/1 -> Add3/1  "theta_c"
  In Bus Element7/1 -> Compute Feed Forward/2(SensorData)
  In Bus Element12/1 -> PID Pitch To Elevator/3
  PID Pitch To Elevator/1 -> Add4/1
  Add3/1 -> PID Pitch To Elevator/1
  Elevator Limit/1 -> dE/1
  [manualMode] -> PID Pitch To Elevator/2
  Add4/1 -> Elevator Limit/1
  In Bus Element14/1 -> Compute Feed Forward/1(dEFFGain)
  [csTrim] -> Selector5/1
  In Bus Element1/1 -> Selector3/1
  reset/1 -> [manualMode]
  ctrlSrfcTrim/1 -> [csTrim]
  Selector3/1 -> Add3/2
  Selector5/1 -> Scope/1, Add4/2
  Compute Feed Forward/1(FF) -> Add4/3

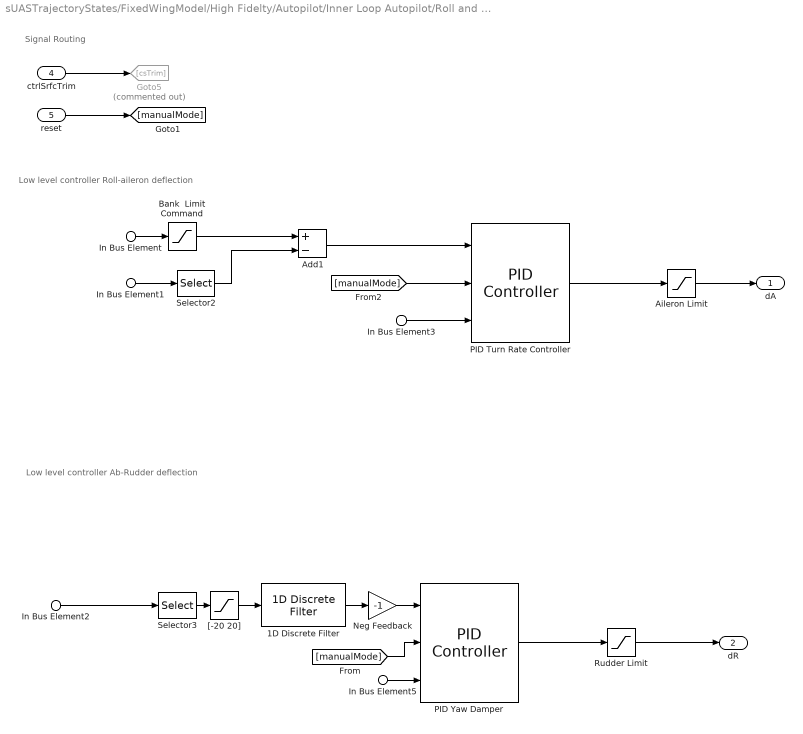
== system sUASTrajectoryStates/FixedWingModel/High Fidelty/Autopilot/Inner Loop Autopilot/Roll and Yaw Controller ==
  note: Signal Routing
  note: Low level controller Ab-Rudder deflection
  note: Low level controller Roll-aileron deflection
  In Bus Element : Inport  PortName=LowLevelCtrlCmds  Element=Roll
  In Bus Element1 : Inport  Port=2  PortName=AutopilotStates  Element=Euler
  In Bus Element2 : Inport  Port=2  PortName=AutopilotStates  Element=Ab
  In Bus Element3 : Inport  Port=3  PortName=apConfigBus  Element=rollControlPID
  In Bus Element5 : Inport  Port=3  PortName=apConfigBus  Element=yawDamperPID
  ctrlSrfcTrim : Inport  Port=4
  reset : Inport  Port=5
  1D Discrete Filter : mbdriLib/Filtering/1D Discrete Filter  bw=10  TSample=ap.apSampleTime
      settings: AttributesFormatString=Fc = 10
  Add1 : Sum  Inputs=+-  OutDataTypeStr=single
  Aileron Limit : Saturate  UpperLimit=ap.control.daLimit  LowerLimit=-ap.control.daLimit
      settings: AttributesFormatString="[%<LowerLimit>  %<UpperLimit>]"
  Bank  Limit Command : Saturate  UpperLimit=ap.control.phi_cLimit  LowerLimit=-ap.control.phi_cLimit
      settings: AttributesFormatString="[%<LowerLimit>  %<UpperLimit>]"
  Goto5 : Goto  Commented=on  GotoTag=csTrim
      settings: AttributesFormatString=[%<GotoTag>]
  Neg Feedback : Gain  Gain=-1  OutDataTypeStr=float('double')
      settings: AttributesFormatString=%<Gain>
  PID Turn Rate Controller : mbdriLib/Control/PID Controller  Tsample=ap.apSampleTime  Ndelay=ap.control.derivativesConstant  upperSaturationLimit=ap.control.daLimit  lowerSaturationLimit=-ap.control.daLimit
  PID Yaw Damper : mbdriLib/Control/PID Controller  Tsample=ap.apSampleTime  Ndelay=ap.control.derivativesConstant  upperSaturationLimit=ap.control.drLimit  lowerSaturationLimit=-ap.control.drLimit
  Rudder Limit : Saturate  UpperLimit=ap.control.drLimit  LowerLimit=-ap.control.drLimit
      settings: AttributesFormatString="[%<LowerLimit>  %<UpperLimit>]"
  Selector2 : Selector  InputPortWidth=3  IndexOptions=Index vector (dialog)  Indices=[1]  OutputSizes=1
  Selector3 : Selector  InputPortWidth=3  IndexOptions=Index vector (dialog)  Indices=[2]  OutputSizes=1
  "[-20 20]" : Saturate  UpperLimit=20  LowerLimit=-20
      settings: AttributesFormatString="[%<LowerLimit>  %<UpperLimit>]"
  dA : Outport  VectorParamsAs1DForOutWhenUnconnected=off
  dR : Outport  Port=2  VectorParamsAs1DForOutWhenUnconnected=off
  wires:
  [manualMode] -> PID Turn Rate Controller/2
  In Bus Element2/1 -> Selector3/1
  Selector3/1 -> "[-20 20]"/1
  [manualMode] -> PID Yaw Damper/2
  In Bus Element5/1 -> PID Yaw Damper/3
  Selector2/1 -> Add1/2
  In Bus Element1/1 -> Selector2/1
  Bank  Limit Command/1 -> Add1/1
  ctrlSrfcTrim/1 -> Goto5/1
  1D Discrete Filter/1 -> Neg Feedback/1
  "[-20 20]"/1 -> 1D Discrete Filter/1
  Neg Feedback/1 -> PID Yaw Damper/1
  In Bus Element/1 -> Bank  Limit Command/1
  Add1/1 -> PID Turn Rate Controller/1
  Aileron Limit/1 -> dA/1
  PID Turn Rate Controller/1 -> Aileron Limit/1
  In Bus Element3/1 -> PID Turn Rate Controller/3
  PID Yaw Damper/1 -> Rudder Limit/1
  Rudder Limit/1 -> dR/1
  reset/1 -> [manualMode]

== system sUASTrajectoryStates/FixedWingModel/High Fidelty/Sensor Module/Position Filter/Baro Altimeter ==
  Static (Pa) : Inport
  Constant : Constant  Value=101325
      settings: AttributesFormatString=%<Value>
  Constant1 : Constant  Value=-8.31432
      settings: AttributesFormatString=%<Value>
  Constant2 : Constant  Value=288.15
      settings: AttributesFormatString=%<Value>
  Constant3 : Constant  Value=0.0289644
      settings: AttributesFormatString=%<Value>
  Constant4 : Constant  Value=env.ISA_g
      settings: AttributesFormatString=%<Value>
  Divide : Product  Inputs=*/
  Math Function : Math  Operator=log  SignedPower=on  SaturateOnIntegerOverflow=on
  Product : Product  Inputs=***//
  "[80k - 120k]" : Saturate  UpperLimit=160000  LowerLimit=80000
      settings: AttributesFormatString="[%<LowerLimit>  %<UpperLimit>]"
  Altitude : Outport  VectorParamsAs1DForOutWhenUnconnected=off
  wires:
  Product/1 -> Altitude/1
  Constant4/1 -> Product/5
  Constant3/1 -> Product/4
  Constant2/1 -> Product/3
  Constant1/1 -> Product/2
  Math Function/1 -> Product/1
  Divide/1 -> Math Function/1
  "[80k - 120k]"/1 -> Divide/1
  Constant/1 -> Divide/2
  Static (Pa)/1 -> "[80k - 120k]"/1

== system sUASTrajectoryStates/FixedWingModel/High Fidelty/Sensor Module/Position Filter/GPS Update ==
  note: If any of the coordinates have changed, set output to 1
  Xe : Inport
  Detect Change : simulink/Logic and Bit Operations/Detect Change  vinit=0  OutDataTypeStr=boolean
  Logical Operator : Logic  Operator=OR  Inputs=1  AllPortsSameDT=off  OutDataTypeStr=boolean
  Update? : Outport  VectorParamsAs1DForOutWhenUnconnected=off
  wires:
  Xe/1 -> Detect Change/1
  Detect Change/1 -> Logical Operator/1
  Logical Operator/1 -> Update?/1

== system sUASTrajectoryStates/FixedWingModel/High Fidelty/Sensor Module/Position Filter/Get Vn Ve ==
  COG : Inport
  SOG : Inport  Port=2
  Angle Conversion : aerolibconvert2/Angle Conversion  IU=deg  OU=rad
  Product : Product  RndMeth=Zero
  Product1 : Product  RndMeth=Zero
  Subsystem5 : Subsystem
  Vnorth : Outport  Unit=m/s  VectorParamsAs1DForOutWhenUnconnected=off
  Veast : Outport  Port=2  Unit=m/s  VectorParamsAs1DForOutWhenUnconnected=off
  wires:
  Product1/1 -> Vnorth/1
  Product/1 -> Veast/1
  SOG/1 -> Product1/1, Product/2
  Angle Conversion/1 -> Subsystem5/1(u)
  Subsystem5/1(sin(u)) -> Product/1
  Subsystem5/2(cos(u)) -> Product1/2
  COG/1 -> Angle Conversion/1

== system sUASTrajectoryStates/FixedWingModel/High Fidelty/Sensor Module/Position Filter/LLA to Flat Earth ==
  latLon : Inport
  h : Inport  Port=2
  COG : Inport  Port=3
  SOG : Inport  Port=4
  initPos : Inport  Port=5
  Enable : EnablePort
  Data Type Conversion : DataTypeConversion  OutDataTypeStr=single
  Data Type Conversion1 : DataTypeConversion  OutDataTypeStr=double
  Data Type Conversion2 : DataTypeConversion  OutDataTypeStr=double
  Data Type Conversion3 : DataTypeConversion  OutDataTypeStr=double
  LLA to Flat Earth : aerolibtransform2/LLA to Flat Earth  units=Metric (MKS)  ptype=Earth (WGS84)  F=1/298.257223563  R=6378137  refPosPort=off  LL0=uavParam.ic.gsLL  psi=0
      settings: SourceProductBaseCode=AE
  Selector : Selector  InputPortWidth=3  IndexOptions=Index vector (dialog)  Indices=[3]  OutputSizes=1
  Xe : Outport  VectorParamsAs1DForOutWhenUnconnected=off
  COG_out : Outport  Port=2  VectorParamsAs1DForOutWhenUnconnected=off
  SOG_out : Outport  Port=3  VectorParamsAs1DForOutWhenUnconnected=off
  wires:
  SOG/1 -> SOG_out/1
  COG/1 -> COG_out/1
  Selector/1 -> Data Type Conversion3/1
  latLon/1 -> Data Type Conversion1/1
  initPos/1 -> Selector/1
  h/1 -> Data Type Conversion2/1
  LLA to Flat Earth/1 -> Data Type Conversion/1
  Data Type Conversion1/1 -> LLA to Flat Earth/1
  Data Type Conversion2/1 -> LLA to Flat Earth/2
  Data Type Conversion3/1 -> LLA to Flat Earth/3
  Data Type Conversion/1 -> Xe/1

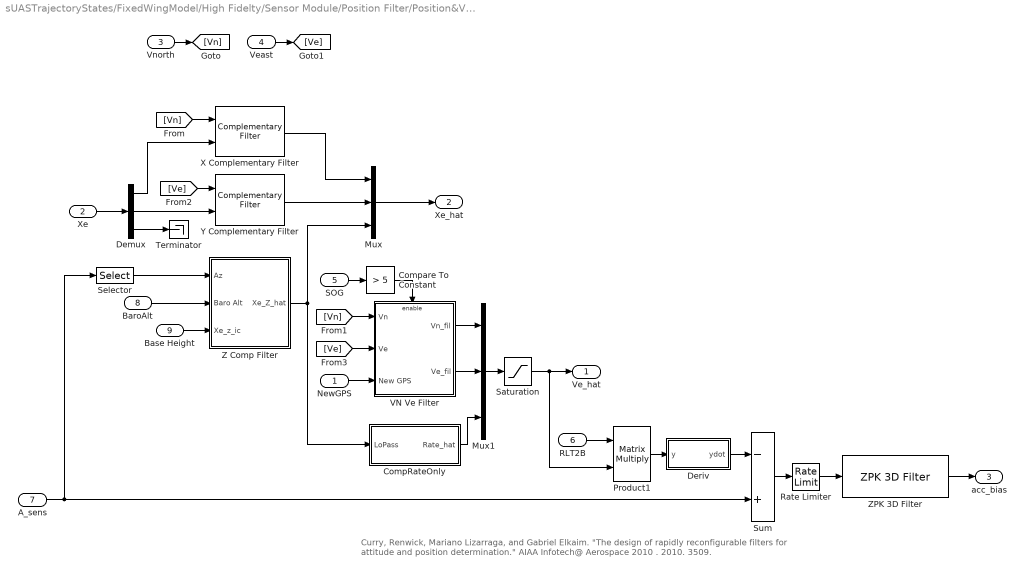
== system sUASTrajectoryStates/FixedWingModel/High Fidelty/Sensor Module/Position Filter/Position&Velocity Filter ==
  note: Curry, Renwick, Mariano Lizarraga, and Gabriel Elkaim. "The design of rapidly reconfigurable filters for attitude and position determination." AIAA Infotech@ Aerospace 2010 . 2010. 3509.
  NewGPS : Inport
  Xe : Inport  Port=2
  Vnorth : Inport  Port=3
  Veast : Inport  Port=4
  SOG : Inport  Port=5
  RLT2B : Inport  Port=6
  A_sens : Inport  Port=7  Unit=m/s^2
  BaroAlt : Inport  Port=8
  Base Height : Inport  Port=9
  CompRateOnly : Subsystem  mask{omega=ap.cf.vzCutoff, T=ap.apSampleTime}
      mask prompts: omega "Cutoff Freq (rad/sec)"; T "Sample Time"
  Compare To Constant : simulink/Logic and Bit Operations/Compare To Constant  relop=>  const=5  OutDataTypeStr=boolean  ZeroCross=off
  Demux : Demux  Outputs=3
  "Deriv " : Subsystem
  Mux : Mux  Inputs=3
  Mux1 : Mux  Inputs=3
  Product1 : Product  Multiplication=Matrix(*)  RndMeth=Zero
  Rate Limiter : RateLimiter  RisingSlewLimit=ap.cf.accBiasRateLimit  FallingSlewLimit=-ap.cf.accBiasRateLimit  SampleTimeMode=inherited
  Saturation : Saturate  UpperLimit=40  LowerLimit=-40
      settings: AttributesFormatString="[%<LowerLimit>  %<UpperLimit>]"
  Selector : Selector  InputPortWidth=3  IndexOptions=Index vector (dialog)  Indices=[3]  OutputSizes=1
  Sum : Sum  Inputs=-+  OutDataTypeStr=single
  Terminator : Terminator
  VN Ve Filter : Subsystem
  X Complementary Filter : mbdriLib/Filtering/Complementary Filter  omega=ap.cf.xCutoff  T=ap.apSampleTime
  Y Complementary Filter : mbdriLib/Filtering/Complementary Filter  omega=ap.cf.yCutoff  T=ap.apSampleTime
  Z Comp Filter : Subsystem
  ZPK 3D Filter : mbdriLib/Filtering/ZPK 3D Filter  zval=[]  pval=-1/ap.cf.accBiasRateLimit  kval=1  TSample=ap.apSampleTime
  Ve_hat : Outport  VectorParamsAs1DForOutWhenUnconnected=off
  Xe_hat : Outport  Port=2  VectorParamsAs1DForOutWhenUnconnected=off
  acc_bias : Outport  Port=3  Unit=m/s^2  VectorParamsAs1DForOutWhenUnconnected=off
  wires:
  Saturation/1 -> Ve_hat/1, Product1/2
  Z Comp Filter/1(Xe_Z_hat) -> Mux/3, CompRateOnly/1(LoPass)
  BaroAlt/1 -> Z Comp Filter/2(Baro Alt)
  Demux/3 -> Terminator/1
  Selector/1 -> Z Comp Filter/1(Az)
  [Ve] -> VN Ve Filter/2(Ve)
  [Ve] -> Y Complementary Filter/1
  Veast/1 -> [Ve]
  [Vn] -> VN Ve Filter/1(Vn)
  [Vn] -> X Complementary Filter/1
  Vnorth/1 -> [Vn]
  CompRateOnly/1(Rate_hat) -> Mux1/3
  VN Ve Filter/2(Ve_fil) -> Mux1/2
  VN Ve Filter/1(Vn_fil) -> Mux1/1
  Mux/1 -> Xe_hat/1
  X Complementary Filter/1 -> Mux/1
  Y Complementary Filter/1 -> Mux/2
  Demux/2 -> Y Complementary Filter/2
  Demux/1 -> X Complementary Filter/2
  Xe/1 -> Demux/1
  Mux1/1 -> Saturation/1
  NewGPS/1 -> VN Ve Filter/3(New GPS)
  Compare To Constant/1 -> VN Ve Filter/Enable
  SOG/1 -> Compare To Constant/1
  Rate Limiter/1 -> ZPK 3D Filter/1
  ZPK 3D Filter/1 -> acc_bias/1
  Sum/1 -> Rate Limiter/1
  Product1/1 -> "Deriv "/1(y)
  "Deriv "/1(ydot) -> Sum/1
  A_sens/1 -> Selector/1, Sum/2
  RLT2B/1 -> Product1/1
  Base Height/1 -> Z Comp Filter/3(Xe_z_ic)

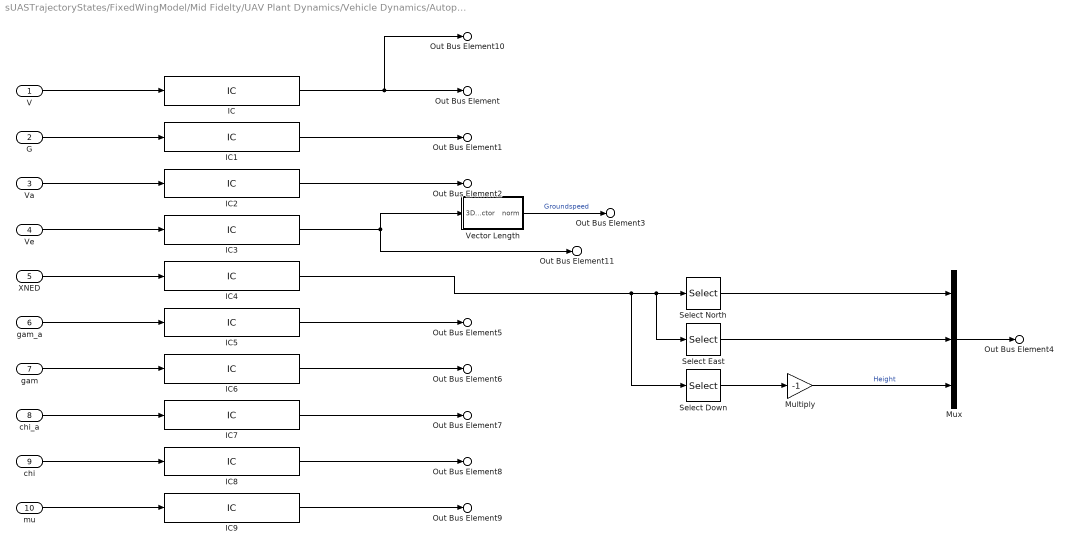
== system sUASTrajectoryStates/FixedWingModel/Mid Fidelty/UAV Plant Dynamics/Vehicle Dynamics/AutopilotStates ==
  V : Inport
  G : Inport  Port=2
  Va : Inport  Port=3
  Ve : Inport  Port=4
  XNED : Inport  Port=5
  gam_a : Inport  Port=6
  gam : Inport  Port=7
  chi_a : Inport  Port=8
  chi : Inport  Port=9
  mu : Inport  Port=10
  IC : InitialCondition  Value=midFidelityUAV.initialAirspeed
  IC1 : InitialCondition  Value=midFidelityUAV.initialAirspeed
  IC2 : InitialCondition  Value=[midFidelityUAV.initialAirspeed 0 0]
  IC3 : InitialCondition  Value=[midFidelityUAV.initialAirspeed 0 0 ]
  IC4 : InitialCondition  Value=[midFidelityUAV.initialNorth midFidelityUAV.initialEast -midFidelityUAV.initialAltitude]
  IC5 : InitialCondition  Value=midFidelityUAV.initialFlightPathAngle
  IC6 : InitialCondition  Value=midFidelityUAV.initialFlightPathAngle
  IC7 : InitialCondition  Value=midFidelityUAV.initialHeadingAngle
  IC8 : InitialCondition  Value=midFidelityUAV.initialHeadingAngle
  IC9 : InitialCondition  Value=0
  Multiply : Gain  Gain=-1
  Mux : Mux  Inputs=3
  Select Down : Selector  InputPortWidth=3  IndexOptions=Index vector (dialog)  Indices=[3]  OutputSizes=1
  Select East : Selector  InputPortWidth=3  IndexOptions=Index vector (dialog)  Indices=[2]  OutputSizes=1
  Select North : Selector  InputPortWidth=3  IndexOptions=Index vector (dialog)  Indices=[1]  OutputSizes=1
  Vector Length : Subsystem
  Out Bus Element : Outport  PortName=AutopilotStates  Element=V
  Out Bus Element1 : Outport  PortName=AutopilotStates  Element=G
  Out Bus Element2 : Outport  PortName=AutopilotStates  Element=Va
  Out Bus Element3 : Outport  PortName=AutopilotStates  Element=GS
  Out Bus Element4 : Outport  PortName=AutopilotStates  Element=Xe
  Out Bus Element5 : Outport  PortName=AutopilotStates  Element=gamma_a
  Out Bus Element6 : Outport  PortName=AutopilotStates  Element=gamma
  Out Bus Element7 : Outport  PortName=AutopilotStates  Element=chi_a
  Out Bus Element8 : Outport  PortName=AutopilotStates  Element=chi
  Out Bus Element9 : Outport  PortName=AutopilotStates  Element=mu
  Out Bus Element10 : Outport  PortName=AutopilotStates  Element=ias
  Out Bus Element11 : Outport  PortName=AutopilotStates  Element=Ve
  wires:
  IC8/1 -> Out Bus Element8/1
  mu/1 -> IC9/1
  Vector Length/1(norm) -> Out Bus Element3/1  "Groundspeed"
  V/1 -> IC/1
  IC/1 -> Out Bus Element/1, Out Bus Element10/1
  G/1 -> IC1/1
  Va/1 -> IC2/1
  Ve/1 -> IC3/1
  XNED/1 -> IC4/1
  gam_a/1 -> IC5/1
  gam/1 -> IC6/1
  chi_a/1 -> IC7/1
  chi/1 -> IC8/1
  IC1/1 -> Out Bus Element1/1
  IC2/1 -> Out Bus Element2/1
  IC3/1 -> Vector Length/1(3DVector), Out Bus Element11/1
  IC4/1 -> Select Down/1, Select East/1, Select North/1
  IC5/1 -> Out Bus Element5/1
  IC6/1 -> Out Bus Element6/1
  IC7/1 -> Out Bus Element7/1
  Select Down/1 -> Multiply/1
  Select North/1 -> Mux/1
  Select East/1 -> Mux/2
  Multiply/1 -> Mux/3  "Height"
  Mux/1 -> Out Bus Element4/1
  IC9/1 -> Out Bus Element9/1
